simulink subsystem "Engine_Map_2WD_NO_REGEN_FILTERED"  (R2023b)
settings: Solver=VariableStepAuto  StartTime=0.0  StopTime=10.0  RelTol=1e-3
undefined symbols (not defined in the file): dK, minK, V, w
settings Model: Creator=Inver  LastModifiedBy=Inver

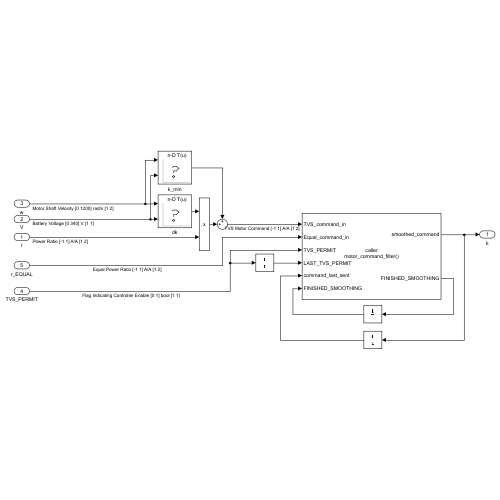
[thumbnail: Simulink's stored preview of the top-level diagram]
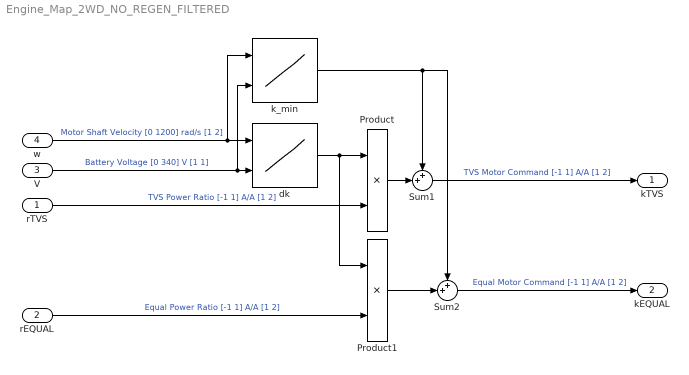
== system Engine_Map_2WD_NO_REGEN_FILTERED ==
  rTVS : Inport
  rEQUAL : Inport  Port=2
  V : Inport  Port=3
  w : Inport  Port=4
  Product : Product
  Product1 : Product
  Sum1 : Sum  Inputs=++|
  Sum2 : Sum  Inputs=++|
  dk : Lookup_n-D  LookupTableObject=''  BreakpointsForDimension1=w  BreakpointsForDimension2=V  BreakpointsForDimension1FirstPoint=10  BreakpointsForDimension2FirstPoint=10  BreakpointsForDimension1Spacing=12  BreakpointsForDimension2Spacing=12  IndexSearchMethod=Evenly spaced points  BeginIndexSearchUsingPreviousIndexResult=on  Table=dK  ExtrapMethod=Clip  RemoveProtectionInput=on  UseLastTableValue=on  InternalRulePriority=Speed  RndMeth=Simplest
      settings: InputPortMap=u0,u1
  k_min : Lookup_n-D  LookupTableObject=''  BreakpointsForDimension1=w  BreakpointsForDimension2=V  BreakpointsForDimension1FirstPoint=10  BreakpointsForDimension2FirstPoint=10  BreakpointsForDimension1Spacing=12  BreakpointsForDimension2Spacing=12  IndexSearchMethod=Evenly spaced points  BeginIndexSearchUsingPreviousIndexResult=on  Table=minK  ExtrapMethod=Clip  RemoveProtectionInput=on  UseLastTableValue=on  InternalRulePriority=Speed  RndMeth=Simplest
      settings: InputPortMap=u0,u1
  kTVS : Outport
  kEQUAL : Outport  Port=2
  wires:
  w/1 -> dk/1, k_min/1  "Motor Shaft Velocity [0 1200] rad/s [1 2]"
  V/1 -> dk/2, k_min/2  "Battery Voltage [0 340] V [1 1]"
  rTVS/1 -> Product/2  "TVS Power Ratio [-1 1] A/A [1 2]"
  Sum1/1 -> kTVS/1  "TVS Motor Command [-1 1] A/A [1 2]"
  k_min/1 -> Sum1/1, Sum2/1
  dk/1 -> Product/1, Product1/1
  Product/1 -> Sum1/2
  rEQUAL/1 -> Product1/2  "Equal Power Ratio [-1 1] A/A [1 2]"
  Product1/1 -> Sum2/2
  Sum2/1 -> kEQUAL/1  "Equal Motor Command [-1 1] A/A [1 2]"
